simulink model "Simulation_V03"  (R2024b)
settings: Solver=VariableStepAuto  StartTime=0.0  StopTime=0.001  FixedStep=0.1e-6  MaxStep=0.001e-6  MinStep=0.0001e-6  RelTol=1e-3
libraries: spsSeriesRLCBranchLib x4, spsMultimeterLib x3, spsCurrentMeasurementLib x2, spsDCVoltageSourceLib x1, spsDiodeLib x1, spsLinearTransformerLib x1, spsMosfetLib x1, sps_lib x1
settings Model: Creator=Mohammad Derogarian  LastModifiedBy=Mohammad Derogarian
settings SolverCC: ZeroCrossAlgorithm=Adaptive
settings DebuggingCC: IgnoredZcDiagnostic=none
settings RTWCC: GPUComputeCapability=3.5

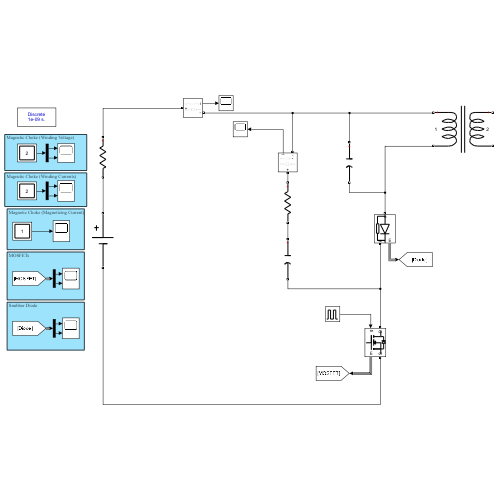
[thumbnail: Simulink's stored preview of the top-level diagram]
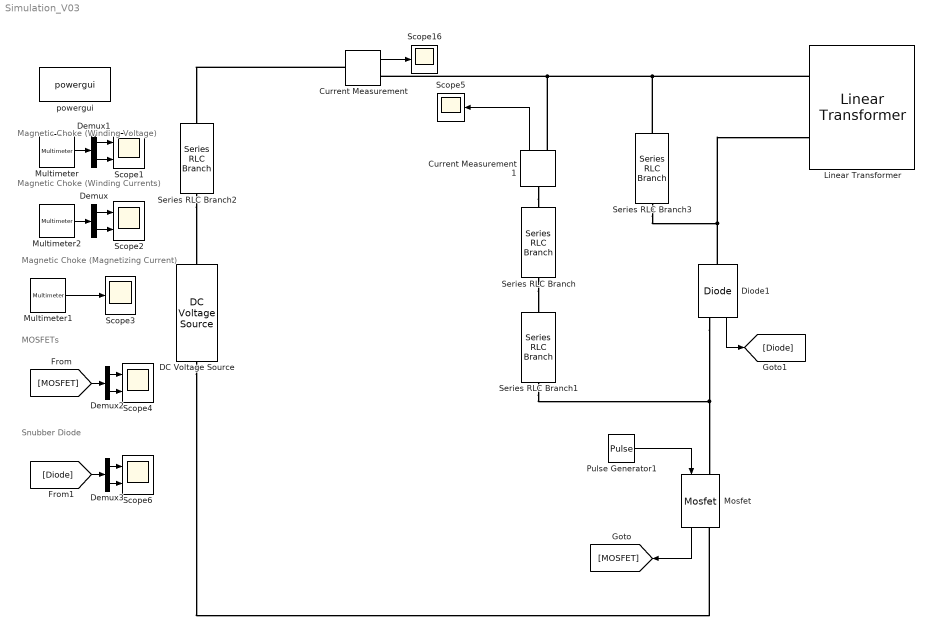
== system Simulation_V03 ==
  note: Magnetic Choke (Winding Voltage)
  note: Magnetic Choke (Winding Currents)
  note: Magnetic Choke (Magnetizing Current)
  note: MOSFETs
  note: Snubber Diode
  Current Measurement : spsCurrentMeasurementLib/Current Measurement  PhasorSimulation=off  OutputType=Complex  PSBequivalent=0
  Current Measurement1 : spsCurrentMeasurementLib/Current Measurement  PhasorSimulation=off  OutputType=Complex  PSBequivalent=0
  DC Voltage Source : spsDCVoltageSourceLib/DC Voltage Source  Amplitude=24  Measurements=None
  Demux{,1..3} (4 alike) : Demux  Outputs=2
  Diode1 : spsDiodeLib/Diode  Ron=0.001  Lon=0  Vf=0.8  IC=0  UseSnubber=0  Rs=500  Cs=250e-9  Measurements=on
  Linear Transformer : spsLinearTransformerLib/Linear Transformer  UNITS=SI  NominalPower=[500 50000 ]  winding1=[30 2 4.5837e-07]  winding2=[1000 4 0.0005093]  ThreeWindings=off  winding3=[3.15e+05 3.969e+05 50.535]  RmLm=[900 10e-6]  Measurements=All voltages and currents  DataType=on
  Mosfet : spsMosfetLib/Mosfet  Ron=0.1  Lon=0  Rd=0.01  Vfd=0  IC=0  Rs=1e5  Cs=inf  Measurements=on
  Multimeter : spsMultimeterLib/Multimeter  L=7  sel=[1 2]  yselected={}  Gain=[1 1]  OutputType=Complex  PlotAtSimulationStop=off  PhasorSimulation=off
  Multimeter1 : spsMultimeterLib/Multimeter  L=7  sel=6  yselected={}  Gain=1  OutputType=Complex  PlotAtSimulationStop=off  PhasorSimulation=off
  Multimeter2 : spsMultimeterLib/Multimeter  L=7  sel=[3 4]  yselected={}  Gain=[1 1]  OutputType=Complex  PlotAtSimulationStop=off  PhasorSimulation=off
  Pulse Generator1 : DiscretePulseGenerator  PulseType=Time based  Period=1/(40e3)  PulseWidth=55
  Scope{1..2,4,6} (4 alike) : Scope  NumInputPorts=2
  Scope16 : Scope
  Scope3 : Scope
  Scope5 : Scope
  Series RLC Branch : spsSeriesRLCBranchLib/Series RLC Branch  LConnTagsString=__new0  RConnTagsString=__new0  BranchType=R  Resistance=1.2e3  Inductance=1e-3  SetiL0=off  InitialCurrent=0  Capacitance=10e-9  Setx0=off  InitialVoltage=0  Measurements=None
  Series RLC Branch1 : spsSeriesRLCBranchLib/Series RLC Branch  LConnTagsString=__new0  RConnTagsString=__new0  BranchType=C  Resistance=1.2e3  Inductance=1e-3  SetiL0=off  InitialCurrent=0  Capacitance=10e-9  Setx0=off  InitialVoltage=0  Measurements=None
  Series RLC Branch2 : spsSeriesRLCBranchLib/Series RLC Branch  LConnTagsString=__new0  RConnTagsString=__new0  BranchType=R  Resistance=1  Inductance=1e-3  SetiL0=off  InitialCurrent=0  Capacitance=10e-9  Setx0=off  InitialVoltage=0  Measurements=None
  Series RLC Branch3 : spsSeriesRLCBranchLib/Series RLC Branch  LConnTagsString=__new0  RConnTagsString=__new0  BranchType=C  Resistance=1.2e3  Inductance=1e-3  SetiL0=off  InitialCurrent=0  Capacitance=1000e-12  Setx0=off  InitialVoltage=0  Measurements=None
  powergui : sps_lib/powergui  Priority=1  SimulationMode=Discrete  SampleTime=0.001e-6  frequency=60  Iterations=50  frequencyindice=0  Pbase=100e6  ErrMax=1e-4  UnitsV=kV  UnitsW=MW  buscounter=0  FunctionMessages=off  echomessages=off  EnableUseOfTLC=off  CurrentSourceSwitches=off  DisableSnubberDevices=off  DisableRonSwitches=off  DisableVfSwitches=off  DisplayEquations=off  AutomaticDiscreteSolvers=off  SolverType=Tustin/Backward Euler (TBE)  Interpol=off  ExternalGateDelay=off  methode=off  Ts=100  x0status=blocks  SPID=on  SwTol=0  HookPort=off  NonlinearTolerance=1e-4  nMaxIteration=100  ContinueOnMaxIteration=off  RestoreLinks=warning  ResistiveCurrentMeasurement=off  Frange=[0:2:500]  Ylog=off  Xlog=on  ShowGrid=off  save=off  variable=ZData  structure=0  ZoomFFT=off  StartTime=0.0  cycles=1  DisplayStyle=1  fundamental=60  FreqAxis=off  MaxFrequency=1000  frequencyindicesteady=1  RmsSteady=1  display=off
  wires:
  Current Measurement/1 -> Scope16/1
  Pulse Generator1/1 -> Mosfet/1
  Demux1/2 -> Scope1/2
  Multimeter2/1 -> Demux/1
  Multimeter/1 -> Demux1/1
  Demux1/1 -> Scope1/1
  Demux/1 -> Scope2/1
  Demux/2 -> Scope2/2
  Multimeter1/1 -> Scope3/1
  Mosfet/1 -> [MOSFET]
  [MOSFET] -> Demux2/1
  Demux2/1 -> Scope4/1
  Demux2/2 -> Scope4/2
  Current Measurement1/1 -> Scope5/1
  Diode1/1 -> [Diode]
  Demux3/2 -> Scope6/2
  Demux3/1 -> Scope6/1
  [Diode] -> Demux3/1
  connections:
  Current Measurement/LConn1 -- Series RLC Branch2/LConn1
  Linear Transformer/LConn1 -- Current Measurement1/RConn1 -- Current Measurement/RConn1 -- Series RLC Branch3/LConn1
  DC Voltage Source/LConn1 -- Mosfet/RConn1
  Diode1/LConn1 -- Series RLC Branch3/RConn1 -- Linear Transformer/LConn2
  Diode1/RConn1 -- Series RLC Branch1/RConn1 -- Mosfet/LConn1
  Series RLC Branch/RConn1 -- Series RLC Branch1/LConn1
  Current Measurement1/LConn1 -- Series RLC Branch/LConn1
  Series RLC Branch2/RConn1 -- DC Voltage Source/RConn1
